simulink library "Springs_Axle2_Interconnected"  (R2025b)
settings: Solver=VariableStepAuto  StartTime=0.0  StopTime=10.0  RelTol=1e-3
libraries: Spring_LeftRight x2
Description:
  | Component of Simscape Vehicle Templates Library
  | 
  | Copyright 2018-2025 The MathWorks, Inc.
settings Model: Creator=smiller  LastModifiedBy=smiller
settings SolverCC: AlgebraicLoopSolver=TrustRegion
settings DataIOCC: ReturnWorkspaceOutputs=off
settings OptimizationCC: ReuseModelBlockBuffer=off
settings DebuggingCC: UnconnectedInputMsg=warning  UnconnectedOutputMsg=warning  UnconnectedLineMsg=warning  ArithmeticOperatorsInVariantConditions=warning
settings ModelReferenceCC: EnableRefExpFcnMdlSchedulingChecks=on
settings SFSimCC: CustomCodeUndefinedFunction=UseInterfaceOnly
settings RTWCC: GPUComputeCapability=3.5  DLArmComputeVersion=19.05

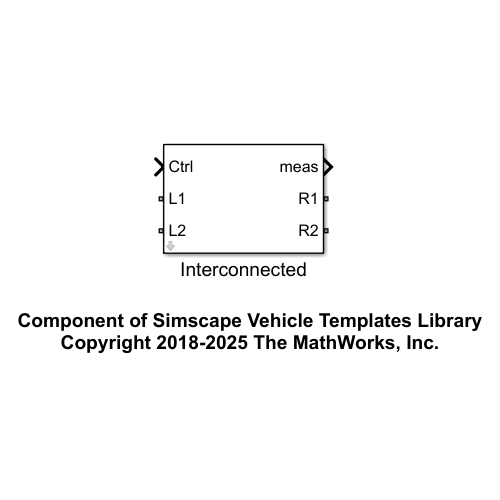
[thumbnail: Simulink's stored preview of the top-level diagram]
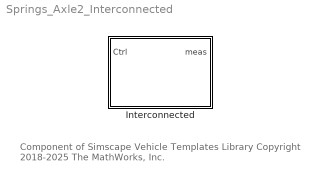
== system Springs_Axle2_Interconnected ==
  note: Component of Simscape Vehicle Templates Library
      | Copyright 2018-2025 The MathWorks, Inc.
  Interconnected : Subsystem  VariantControl=Interconnected  mask(Interconnected Springs){}
      mask help: Springs with connection across left and right sides.

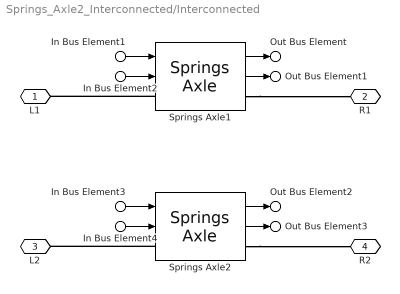
== system Springs_Axle2_Interconnected/Interconnected ==
  In Bus Element1 : Inport  PortName=Ctrl  Element=L1
  In Bus Element2 : Inport  PortName=Ctrl  Element=R1
  In Bus Element3 : Inport  PortName=Ctrl  Element=L2
  In Bus Element4 : Inport  PortName=Ctrl  Element=R2
  Springs Axle1 : Spring_LeftRight/Springs Axle  VariantControl=Variant1  LabelModeActiveChoice=Linear  Spring=Spring.Axle1  VariantLabel=Spring.Axle1.class.Value
      settings: AttributesFormatString=%<ActiveVariant>
  Springs Axle2 : Spring_LeftRight/Springs Axle  VariantControl=Variant1  LabelModeActiveChoice=Linear  Spring=Spring.Axle2  VariantLabel=Spring.Axle2.class.Value
      settings: AttributesFormatString=%<ActiveVariant>
  L1 : PMIOPort  Side=Left
  R1 : PMIOPort  Port=2  Side=Right
  L2 : PMIOPort  Port=3  Side=Left
  R2 : PMIOPort  Port=4  Side=Right
  Out Bus Element : Outport  VectorParamsAs1DForOutWhenUnconnected=off  PortName=meas  Element=L1
  Out Bus Element1 : Outport  VectorParamsAs1DForOutWhenUnconnected=off  PortName=meas  Element=R1
  Out Bus Element2 : Outport  VectorParamsAs1DForOutWhenUnconnected=off  PortName=meas  Element=L2
  Out Bus Element3 : Outport  VectorParamsAs1DForOutWhenUnconnected=off  PortName=meas  Element=R2
  wires:
  Springs Axle1/1 -> Out Bus Element/1
  Springs Axle1/2 -> Out Bus Element1/1
  In Bus Element2/1 -> Springs Axle1/2
  In Bus Element1/1 -> Springs Axle1/1
  Springs Axle2/2 -> Out Bus Element3/1
  Springs Axle2/1 -> Out Bus Element2/1
  In Bus Element4/1 -> Springs Axle2/2
  In Bus Element3/1 -> Springs Axle2/1
  connections:
  Springs Axle1/RConn1 -- R1/RConn1
  Springs Axle1/LConn1 -- L1/RConn1
  Springs Axle2/LConn1 -- L2/RConn1
  Springs Axle2/RConn1 -- R2/RConn1
